simulink model "StateFlowChart"  (R2022a)
settings: Solver=VariableStepAuto  StartTime=0.0  StopTime=10.0  RelTol=1e-3
settings Model: Creator=uie82234  LastModifiedBy=uie82234

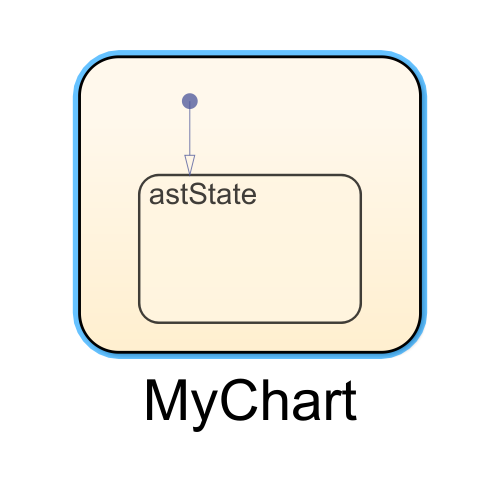
[thumbnail: Simulink's stored preview of the top-level diagram]
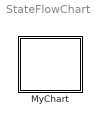
== system StateFlowChart ==
  MyChart : Stateflow chart  TreatAsAtomicUnit=on

== stateflow chart StateFlowChart/MyChart ==
  state astState
  (default) -> astState
